simulink model "parte1_pert_carga_discrete"  (R2021b)
settings: Solver=VariableStepAuto  StartTime=0.0  StopTime=6  RelTol=1e-3
values from neighbouring files (symbols this model uses):
  h = 0.03    [parte1_script.m]
  Jm = 1.3475e-6    (= 1.3475e-06)    [parte1_script.m]
  Ke = 0.0159    [parte1_script.m]
  Kf = 0.000001176    (= 1.176e-06)    [parte1_script.m]
  Ki = wn^2 / K1    [parte1_script.m]
  Kp = (2*zeta*wn -alfa)/K1    [parte1_script.m]
  La = 0    [parte1_script.m]
  Ra = 8    [parte1_script.m]
undefined symbols (not defined in the file or in its folder): DiscIntNeverNeededParam
settings Model: Creator=Dylan  LastModifiedBy=Dylan

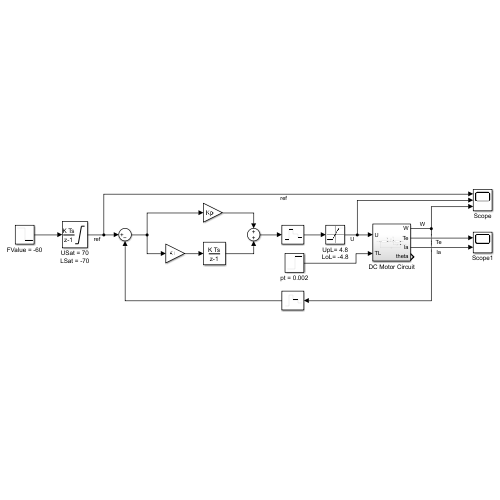
[thumbnail: Simulink's stored preview of the top-level diagram]
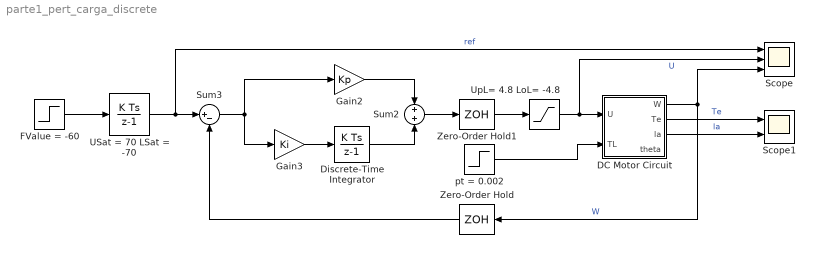
== system parte1_pert_carga_discrete ==
  DC Motor Circuit : Subsystem
  Discrete-Time Integrator : DiscreteIntegrator  SampleTime=h  ICPrevOutput=DiscIntNeverNeededParam  ICPrevScaledInput=DiscIntNeverNeededParam
  FValue = -60 : Step  After=-60  SampleTime=0
  Gain2 : Gain  Gain=Kp
  Gain3 : Gain  Gain=Ki
  Scope : Scope  NumInputPorts=3
  Scope1 : Scope  NumInputPorts=2
  Sum2 : Sum  Inputs=+|+
  Sum3 : Sum  Inputs=|+-
  USat = 70 LSat = -70 : DiscreteIntegrator  SampleTime=h  LimitOutput=on  UpperSaturationLimit=70  LowerSaturationLimit=-70  ICPrevOutput=DiscIntNeverNeededParam  ICPrevScaledInput=DiscIntNeverNeededParam
  UpL= 4.8 LoL= -4.8 : Saturate  UpperLimit=4.8  LowerLimit=-4.8
  Zero-Order Hold : ZeroOrderHold  SampleTime=h
  Zero-Order Hold1 : ZeroOrderHold  SampleTime=h
  pt = 0.002 : Step  Time=5  After=0.002  SampleTime=0
  wires:
  Gain2/1 -> Sum2/1
  UpL= 4.8 LoL= -4.8/1 -> Scope/2, DC Motor Circuit/1(U)  "U"
  DC Motor Circuit/1(W) -> Zero-Order Hold/1, Scope/3  "W"
  Discrete-Time Integrator/1 -> Sum2/2
  pt = 0.002/1 -> DC Motor Circuit/2(TL)
  Sum3/1 -> Gain2/1, Gain3/1
  Gain3/1 -> Discrete-Time Integrator/1
  Zero-Order Hold/1 -> Sum3/2
  Sum2/1 -> Zero-Order Hold1/1
  Zero-Order Hold1/1 -> UpL= 4.8 LoL= -4.8/1
  USat = 70 LSat = -70/1 -> Scope/1, Sum3/1  "ref"
  FValue = -60/1 -> USat = 70 LSat = -70/1
  DC Motor Circuit/2(Te) -> Scope1/1  "Te"
  DC Motor Circuit/3(la) -> Scope1/2  "la"

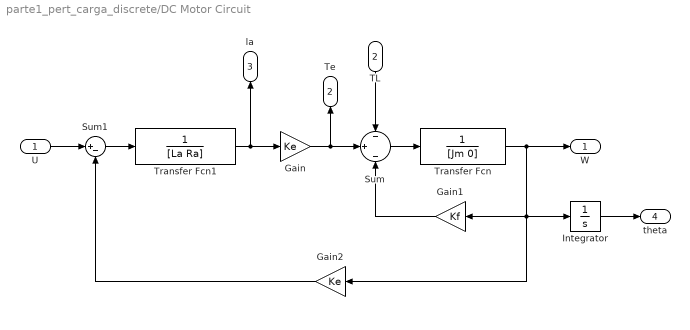
== system parte1_pert_carga_discrete/DC Motor Circuit ==
  U : Inport
  TL : Inport  Port=2
  Gain : Gain  Gain=Ke
  Gain1 : Gain  Gain=Kf
  Gain2 : Gain  Gain=Ke
  Integrator : Integrator
  Sum : Sum  Inputs=-|+|-
  Sum1 : Sum  Inputs=|+-
  Transfer Fcn : TransferFcn  Denominator=[Jm 0]
  Transfer Fcn1 : TransferFcn  Denominator=[La Ra]
  W : Outport
  Te : Outport  Port=2
  la : Outport  Port=3
  theta : Outport  Port=4
  wires:
  U/1 -> Sum1/1
  Transfer Fcn/1 -> W/1, Gain2/1, Integrator/1, Gain1/1
  Transfer Fcn1/1 -> la/1, Gain/1
  Gain2/1 -> Sum1/2
  Sum/1 -> Transfer Fcn/1
  Gain/1 -> Te/1, Sum/2
  TL/1 -> Sum/1
  Gain1/1 -> Sum/3
  Sum1/1 -> Transfer Fcn1/1
  Integrator/1 -> theta/1
